simulink model "BF_Vitesse_22_10_2025"  (R2025a)
settings: Solver=VariableStepAuto  StartTime=0.0  StopTime=0.1  FixedStep=1e-4  RelTol=1e-3
undefined symbols (not defined in the file): J, Kphi, L, R, Rch, U
settings Model: Creator=ltroullier01  LastModifiedBy=ltroullier01

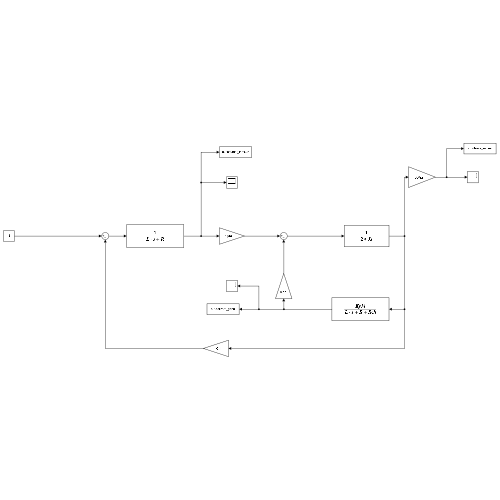
[thumbnail: Simulink's stored preview of the top-level diagram]
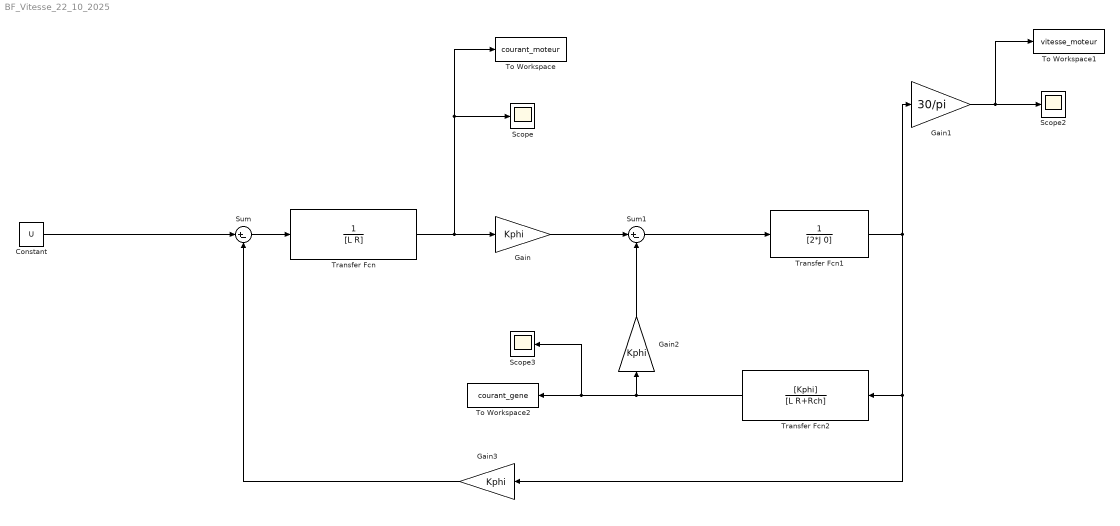
== system BF_Vitesse_22_10_2025 ==
  Constant : Constant  Value=U
  Gain : Gain  Gain=Kphi
  Gain1 : Gain  Gain=30/pi
  Gain2 : Gain  Gain=Kphi
  Gain3 : Gain  Gain=Kphi
  Scope : Scope
      settings: ActiveDisplayYMinimum=-4.9369832712561159  ActiveDisplayYMaximum=31.373841687864346
  Scope2 : Scope
      settings: ActiveDisplayYMinimum=-1903.7496929081253  ActiveDisplayYMaximum=5096.5030674299223  DataLoggingVariableName=ScopeData2
  Scope3 : Scope
      settings: ActiveDisplayYMinimum=-4.9369832712561159  ActiveDisplayYMaximum=31.373841687864346  DataLoggingVariableName=ScopeData3
  Sum : Sum  Inputs=|+-
  Sum1 : Sum  Inputs=|+-
  To Workspace : ToWorkspace  VariableName=courant_moteur  SaveFormat=Timeseries  SampleTime=-1
  To Workspace1 : ToWorkspace  VariableName=vitesse_moteur  SaveFormat=Timeseries  SampleTime=-1
  To Workspace2 : ToWorkspace  VariableName=courant_gene  SaveFormat=Timeseries  SampleTime=-1
  Transfer Fcn : TransferFcn  Denominator=[L R]
  Transfer Fcn1 : TransferFcn  Denominator=[2*J 0]
  Transfer Fcn2 : TransferFcn  Numerator=[Kphi]  Denominator=[L R+Rch]
  wires:
  Constant/1 -> Sum/1
  Sum/1 -> Transfer Fcn/1
  Transfer Fcn1/1 -> Gain3/1, Transfer Fcn2/1, Gain1/1
  Gain1/1 -> To Workspace1/1, Scope2/1
  Transfer Fcn/1 -> To Workspace/1, Scope/1, Gain/1
  Gain/1 -> Sum1/1
  Sum1/1 -> Transfer Fcn1/1
  Gain2/1 -> Sum1/2
  Transfer Fcn2/1 -> Scope3/1, To Workspace2/1, Gain2/1
  Gain3/1 -> Sum/2
